simulink model "servocontrol"  (R2016b)
settings: Solver=VariableStepAuto  StartTime=0.0  StopTime=5  MaxStep=0.01  RelTol=1e-4  EnableMultiTasking=on
values from neighbouring files (symbols this model uses):
  A1 = [ ... (first row only)    [physical_para.m]
  B1 = [ ... (first row only)    [physical_para.m]
  C1 = eye(4)    [physical_para.m]
  C_psi = [0 1 0 0]    [physical_para.m]
  C_theta = [1 0 0 0]    [physical_para.m]
  D1 = zeros(4, 2)    [physical_para.m]
  k_f = KK(:, 1:4)    [physical_para.m]
  k_i = KK(:, 5)    [physical_para.m]
settings Model: Creator=DeLL  LastModifiedBy=DeLL
settings DataIOCC: LimitDataPoints=on  SaveOutput=off  SaveTime=off
settings OptimizationCC: ExpressionDepthLimit=2147483647  LifeSpan=1
settings DebuggingCC: UnderspecifiedInitializationDetection=Classic  MergeDetectMultiDrivingBlocksExec=none  FcnCallInpInsideContextMsg=warning  AllowSymbolicDim=off  StateNameClashWarn=warning  SFUnexpectedBacktrackingDiag=warning  SFNoUnconditionalDefaultTransitionDiag=warning  SFExecutionAtInitializationDiag=none
settings GRTTargetCC: TargetLangStandard=C89/C90 (ANSI)  GeneratePreprocessorConditionals=Disable all  CombineOutputUpdateFcns=off  GRTInterface=on

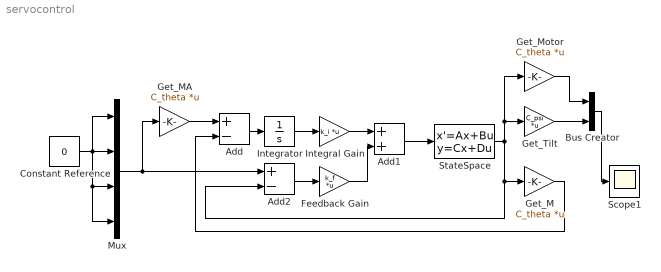
== system servocontrol ==
  Add : Sum  Inputs=+-
  Add1 : Sum
  Add2 : Sum  Inputs=+-
  Bus Creator : BusCreator  Inputs=2
  Constant Reference : Constant  Value=0
  Feedback Gain : Gain  Gain=k_f  Multiplication=Matrix(K*u)
  Get_M : Gain  Gain=C_theta  Multiplication=Matrix(K*u)
  Get_MA : Gain  Gain=C_theta  Multiplication=Matrix(K*u)
  Get_Motor : Gain  Gain=C_theta  Multiplication=Matrix(K*u)
  Get_Tilt : Gain  Gain=C_psi  Multiplication=Matrix(K*u)
  Integral Gain : Gain  Gain=k_i  Multiplication=Matrix(K*u)
  Integrator : Integrator
  Mux : Mux
  Scope1 : Scope
  StateSpace : StateSpace  A=A1  B=B1  C=C1  D=D1  X0=[5 0 0 0]
  wires:
  Add1/1 -> StateSpace/1
  Integral Gain/1 -> Add1/1
  Integrator/1 -> Integral Gain/1
  Add/1 -> Integrator/1
  Get_MA/1 -> Add/1
  Add2/1 -> Feedback Gain/1
  Get_M/1 -> Add/2
  Mux/1 -> Get_MA/1, Add2/1
  Feedback Gain/1 -> Add1/2
  Constant Reference/1 -> Mux/4, Mux/3, Mux/2, Mux/1
  StateSpace/1 -> Get_M/1, Add2/2, Get_Motor/1, Get_Tilt/1
  Get_Tilt/1 -> Bus Creator/2
  Get_Motor/1 -> Bus Creator/1
  Bus Creator/1 -> Scope1/1
